simulink model "Integrated_Model"  (R2022a)
settings: Solver=VariableStepAuto  StartTime=0.0  StopTime=10.0  RelTol=1e-3
libraries: simulink x74, simulink_extras x1
settings Model: Creator=user  LastModifiedBy=hp

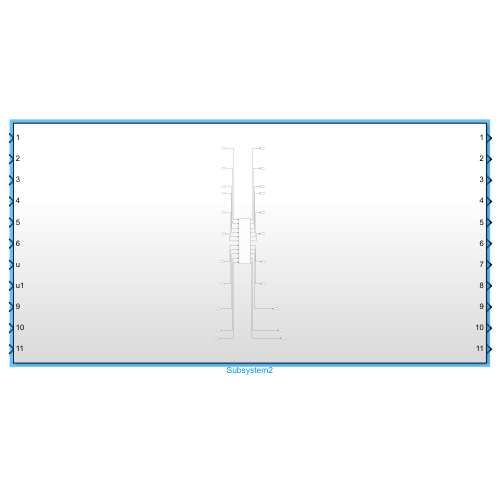
[thumbnail: Simulink's stored preview of the top-level diagram]
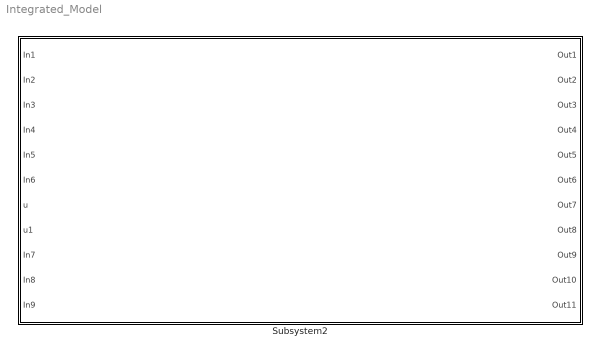
== system Integrated_Model ==
  Subsystem2 : Subsystem

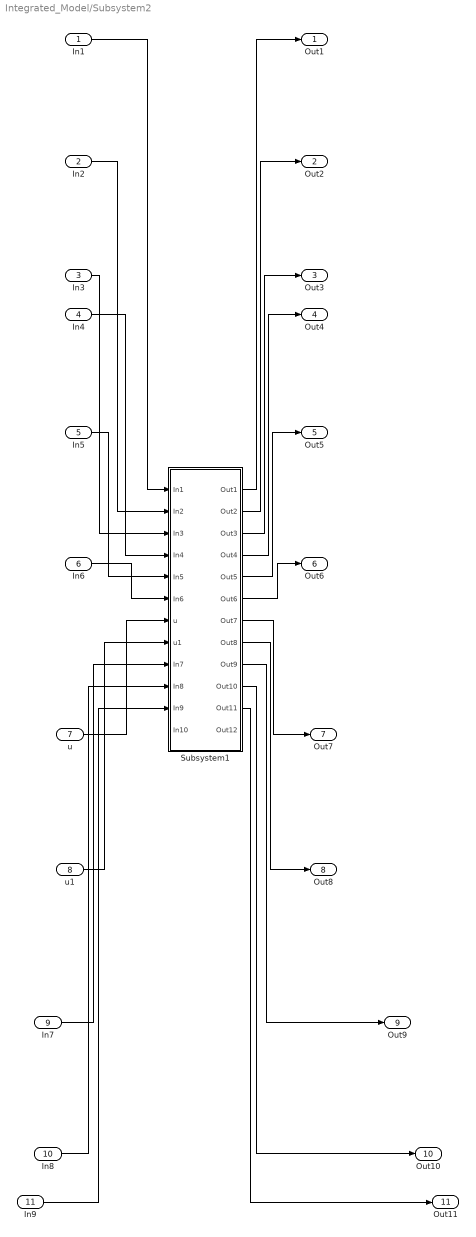
== system Integrated_Model/Subsystem2 ==
  In1 : Inport
  In2 : Inport  Port=2
  In3 : Inport  Port=3
  In4 : Inport  Port=4
  In5 : Inport  Port=5
  In6 : Inport  Port=6
  u : Inport  Port=7
  u1 : Inport  Port=8
  In7 : Inport  Port=9
  In8 : Inport  Port=10
  In9 : Inport  Port=11
  Subsystem1 : Subsystem
  Out1 : Outport
  Out2 : Outport  Port=2
  Out3 : Outport  Port=3
  Out4 : Outport  Port=4
  Out5 : Outport  Port=5
  Out6 : Outport  Port=6
  Out7 : Outport  Port=7
  Out8 : Outport  Port=8
  Out9 : Outport  Port=9
  Out10 : Outport  Port=10
  Out11 : Outport  Port=11
  wires:
  In1/1 -> Subsystem1/1(In1)
  In2/1 -> Subsystem1/2(In2)
  In3/1 -> Subsystem1/3(In3)
  In4/1 -> Subsystem1/4(In4)
  In5/1 -> Subsystem1/5(In5)
  In6/1 -> Subsystem1/6(In6)
  u/1 -> Subsystem1/7(u)
  u1/1 -> Subsystem1/8(u1)
  In7/1 -> Subsystem1/9(In7)
  In8/1 -> Subsystem1/10(In8)
  In9/1 -> Subsystem1/11(In9)
  Subsystem1/1(Out1) -> Out1/1
  Subsystem1/2(Out2) -> Out2/1
  Subsystem1/3(Out3) -> Out3/1
  Subsystem1/4(Out4) -> Out4/1
  Subsystem1/5(Out5) -> Out5/1
  Subsystem1/6(Out6) -> Out6/1
  Subsystem1/7(Out7) -> Out7/1
  Subsystem1/8(Out8) -> Out8/1
  Subsystem1/9(Out9) -> Out9/1
  Subsystem1/10(Out10) -> Out10/1
  Subsystem1/11(Out11) -> Out11/1

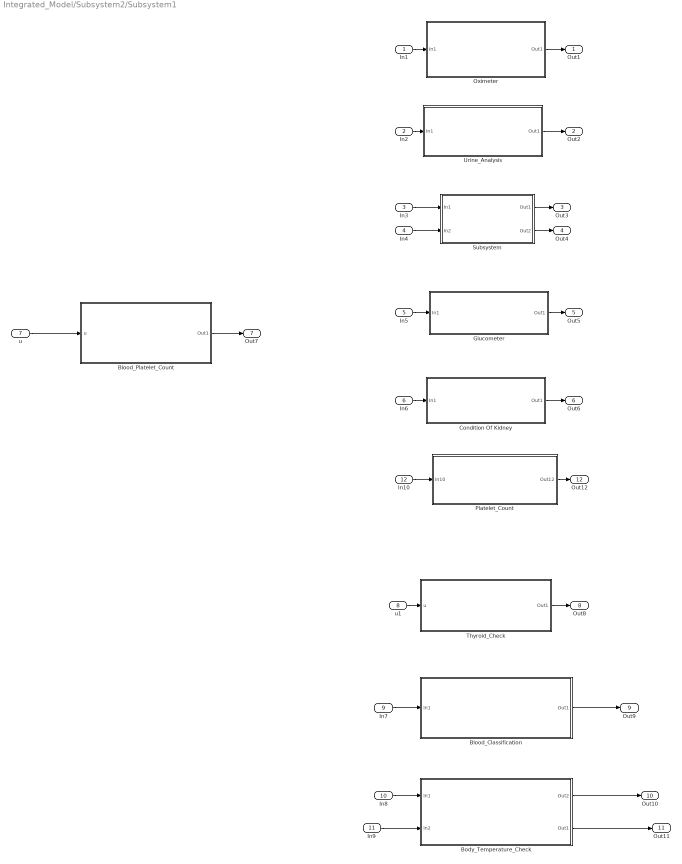
== system Integrated_Model/Subsystem2/Subsystem1 ==
  In1 : Inport
  In2 : Inport  Port=2
  In3 : Inport  Port=3
  In4 : Inport  Port=4
  In5 : Inport  Port=5
  In6 : Inport  Port=6
  u : Inport  Port=7
  u1 : Inport  Port=8
  In7 : Inport  Port=9
  In8 : Inport  Port=10
  In9 : Inport  Port=11
  In10 : Inport  Port=12
  Blood_Classification : Subsystem
  Blood_Platelet_Count : Subsystem
  Body_Temperature_Check : Subsystem
  Condition Of Kidney : Subsystem
  Glucometer : Subsystem
  Oximeter : Subsystem
  Platelet_Count : Subsystem
  Subsystem : Subsystem
  Thyroid_Check : Subsystem
  Urine_Analysis : Subsystem
  Out1 : Outport
  Out2 : Outport  Port=2
  Out3 : Outport  Port=3
  Out4 : Outport  Port=4
  Out5 : Outport  Port=5
  Out6 : Outport  Port=6
  Out7 : Outport  Port=7
  Out8 : Outport  Port=8
  Out9 : Outport  Port=9
  Out10 : Outport  Port=10
  Out11 : Outport  Port=11
  Out12 : Outport  Port=12
  wires:
  In6/1 -> Condition Of Kidney/1(In1)
  Body_Temperature_Check/1(Out2) -> Out10/1
  In8/1 -> Body_Temperature_Check/1(In1)
  In3/1 -> Subsystem/1(In1)
  In4/1 -> Subsystem/2(In2)
  In7/1 -> Blood_Classification/1(In1)
  u1/1 -> Thyroid_Check/1(u)
  In1/1 -> Oximeter/1(In1)
  u/1 -> Blood_Platelet_Count/1(u)
  Urine_Analysis/1(Out1) -> Out2/1
  Subsystem/1(Out1) -> Out3/1
  Subsystem/2(Out2) -> Out4/1
  Oximeter/1(Out1) -> Out1/1
  In2/1 -> Urine_Analysis/1(In1)
  Body_Temperature_Check/2(Out1) -> Out11/1
  Thyroid_Check/1(Out1) -> Out8/1
  Condition Of Kidney/1(Out1) -> Out6/1
  Blood_Classification/1(Out1) -> Out9/1
  Blood_Platelet_Count/1(Out1) -> Out7/1
  In5/1 -> Glucometer/1(In1)
  Glucometer/1(Out1) -> Out5/1
  In9/1 -> Body_Temperature_Check/2(In2)
  In10/1 -> Platelet_Count/1(In10)
  Platelet_Count/1(Out12) -> Out12/1

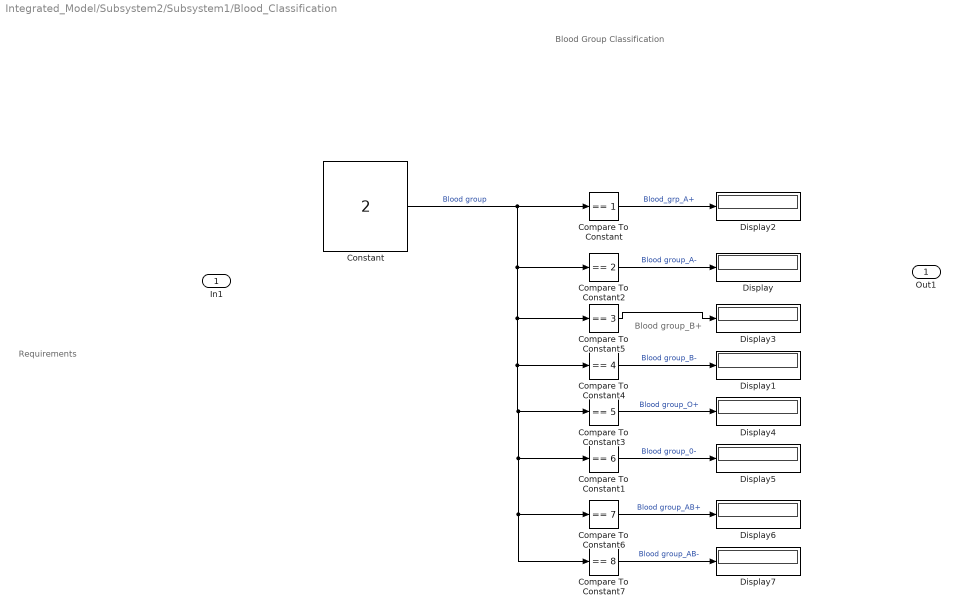
== system Integrated_Model/Subsystem2/Subsystem1/Blood_Classification ==
  note: Requirements
  note: Blood group_B+
  note: Blood Group Classification
  In1 : Inport
  Compare To Constant : simulink/Logic and Bit Operations/Compare To Constant  relop===  const=1  OutDataTypeStr=boolean
  Compare To Constant1 : simulink/Logic and Bit Operations/Compare To Constant  relop===  const=6  OutDataTypeStr=boolean
  Compare To Constant2 : simulink/Logic and Bit Operations/Compare To Constant  relop===  const=2  OutDataTypeStr=boolean
  Compare To Constant3 : simulink/Logic and Bit Operations/Compare To Constant  relop===  const=5  OutDataTypeStr=boolean
  Compare To Constant4 : simulink/Logic and Bit Operations/Compare To Constant  relop===  const=4  OutDataTypeStr=boolean
  Compare To Constant5 : simulink/Logic and Bit Operations/Compare To Constant  relop===  const=3  OutDataTypeStr=boolean
  Compare To Constant6 : simulink/Logic and Bit Operations/Compare To Constant  relop===  const=7  OutDataTypeStr=boolean
  Compare To Constant7 : simulink/Logic and Bit Operations/Compare To Constant  relop===  const=8  OutDataTypeStr=boolean
  Constant : Constant  Value=2
  Display{,1..7} (8 alike) : Display
  Out1 : Outport
  wires:
  Compare To Constant5/1 -> Display3/1
  Compare To Constant4/1 -> Display1/1  "Blood group_B-"
  Constant/1 -> Compare To Constant7/1, Compare To Constant6/1, Compare To Constant1/1, Compare To Constant3/1, Compare To Constant4/1, Compare To Constant5/1, Compare To Constant2/1, Compare To Constant/1  "Blood group"
  Compare To Constant6/1 -> Display6/1  "Blood group_AB+"
  Compare To Constant1/1 -> Display5/1  "Blood group_0-"
  Compare To Constant/1 -> Display2/1  "Blood_grp_A+"
  Compare To Constant2/1 -> Display/1  "Blood group_A-"
  Compare To Constant3/1 -> Display4/1  "Blood group_O+"
  Compare To Constant7/1 -> Display7/1  "Blood group_AB-"

== system Integrated_Model/Subsystem2/Subsystem1/Blood_Platelet_Count ==
  note: BLOOD PLATELET COUNT
  note: INPUTS
      |
      | 0- <150000 Platelets
      | 1- 150000-450000
      | 2- >450000 Platelets
      |
      | OUTPUTS
      | 0 - Thrombocytopenia
      | 1-  Normal
      | 2-  Thrombocytosis
  u : Inport
  Compare To Constant : simulink/Logic and Bit Operations/Compare To Constant  relop===  const=0  OutDataTypeStr=boolean
  Compare To Constant1 : simulink/Logic and Bit Operations/Compare To Constant  relop===  const=1  OutDataTypeStr=boolean
  Compare To Constant2 : simulink/Logic and Bit Operations/Compare To Constant  relop===  const=2  OutDataTypeStr=boolean
  Constant1 : Constant  Value=0
  Constant2 : Constant
  Constant3 : Constant  Value=2
  Constant4 : Constant  Value=2
  Switch : Switch  Criteria=u2 ~= 0  SaturateOnIntegerOverflow=off  InputSameDT=off
  Switch1 : Switch  Criteria=u2 ~= 0  SaturateOnIntegerOverflow=off  InputSameDT=off
  Switch2 : Switch  SaturateOnIntegerOverflow=off  InputSameDT=off
  Out1 : Outport
  wires:
  Switch/1 -> Out1/1
  Constant2/1 -> Switch1/1
  Constant4/1 -> Switch2/3
  Compare To Constant/1 -> Switch/2
  Constant1/1 -> Switch/1
  Compare To Constant2/1 -> Switch2/2
  Compare To Constant1/1 -> Switch1/2
  Switch2/1 -> Switch1/3
  Constant3/1 -> Switch2/1
  Switch1/1 -> Switch/3
  u/1 -> Compare To Constant2/1, Compare To Constant1/1, Compare To Constant/1

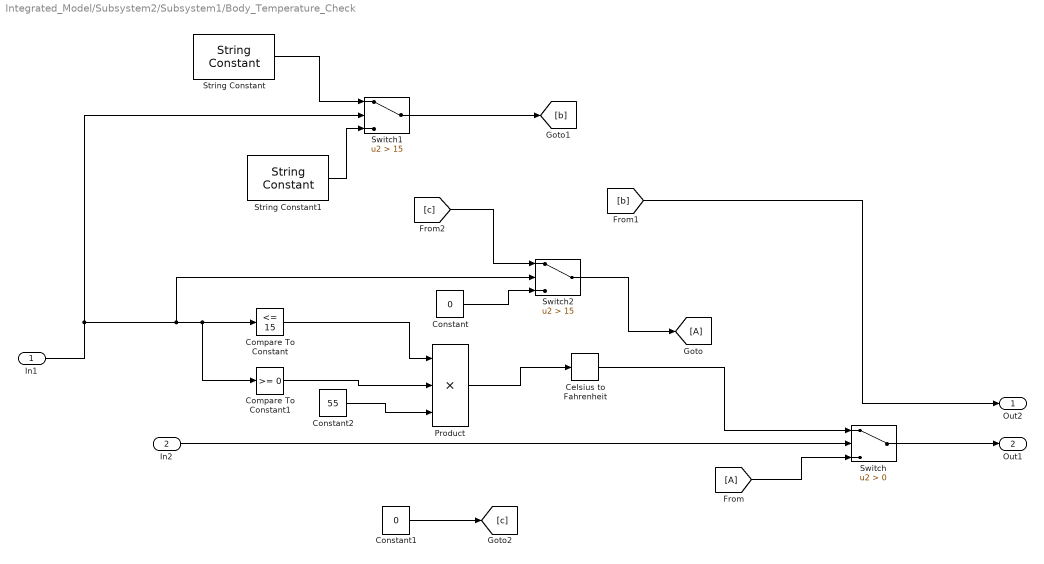
== system Integrated_Model/Subsystem2/Subsystem1/Body_Temperature_Check ==
  In1 : Inport
  In2 : Inport  Port=2
  Celsius to Fahrenheit : simulink_extras/Transformations/Celsius to Fahrenheit
      settings: SourceProductBaseCode=SL
  Compare To Constant : simulink/Logic and Bit Operations/Compare To Constant  relop=<=  const=15  OutDataTypeStr=boolean
  Compare To Constant1 : simulink/Logic and Bit Operations/Compare To Constant  relop=>=  const=0  OutDataTypeStr=boolean
  Constant : Constant  Value=0
  Constant1 : Constant  Value=0
  Constant2 : Constant  Value=55
  From : From
  Goto : Goto
  Product : Product  Inputs=3
  String Constant : StringConstant  String="\"invalid\""
  String Constant1 : StringConstant  String="\"working\""
  Switch : Switch  Criteria=u2 > Threshold  SaturateOnIntegerOverflow=off  InputSameDT=off
  Switch1 : Switch  Criteria=u2 > Threshold  Threshold=15  SaturateOnIntegerOverflow=off  InputSameDT=off
  Switch2 : Switch  Criteria=u2 > Threshold  Threshold=15  SaturateOnIntegerOverflow=off  InputSameDT=off
  Out2 : Outport
  Out1 : Outport  Port=2
  wires:
  Product/1 -> Celsius to Fahrenheit/1
  In2/1 -> Switch/2
  Switch/1 -> Out1/1
  Celsius to Fahrenheit/1 -> Switch/1
  From/1 -> Switch/3
  Constant2/1 -> Product/3
  Compare To Constant/1 -> Product/1
  Compare To Constant1/1 -> Product/2
  String Constant/1 -> Switch1/1
  Switch1/1 -> [b]
  [b] -> Out2/1
  String Constant1/1 -> Switch1/3
  In1/1 -> Switch2/2, Compare To Constant1/1, Compare To Constant/1, Switch1/2
  Switch2/1 -> Goto/1
  Constant/1 -> Switch2/3
  [c] -> Switch2/1
  Constant1/1 -> [c]

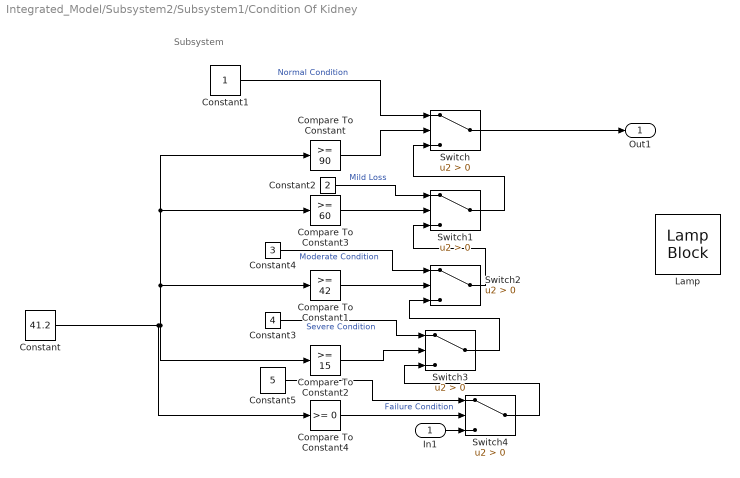
== system Integrated_Model/Subsystem2/Subsystem1/Condition Of Kidney ==
  note: Subsystem
  In1 : Inport
  Compare To Constant : simulink/Logic and Bit Operations/Compare To Constant  relop=>=  const=90  OutDataTypeStr=boolean
  Compare To Constant1 : simulink/Logic and Bit Operations/Compare To Constant  relop=>=  const=42  OutDataTypeStr=boolean
  Compare To Constant2 : simulink/Logic and Bit Operations/Compare To Constant  relop=>=  const=15  OutDataTypeStr=boolean
  Compare To Constant3 : simulink/Logic and Bit Operations/Compare To Constant  relop=>=  const=60  OutDataTypeStr=boolean
  Compare To Constant4 : simulink/Logic and Bit Operations/Compare To Constant  relop=>=  const=0  OutDataTypeStr=boolean
  Constant : Constant  Value=41.2
  Constant1 : Constant
  Constant2 : Constant  Value=2
  Constant3 : Constant  Value=4
  Constant4 : Constant  Value=3
  Constant5 : Constant  Value=5
  Lamp : LampBlock  LabelPosition=Hide
  Switch{,1..4} (5 alike) : Switch  Criteria=u2 > Threshold  SaturateOnIntegerOverflow=off  InputSameDT=off
  Out1 : Outport
  wires:
  Compare To Constant/1 -> Switch/2
  Constant1/1 -> Switch/1  "Normal Condition"
  Compare To Constant4/1 -> Switch4/2
  Switch2/1 -> Switch1/3
  Constant/1 -> Compare To Constant3/1, Compare To Constant/1, Compare To Constant1/1, Compare To Constant2/1, Compare To Constant4/1
  Switch4/1 -> Switch3/3
  Switch1/1 -> Switch/3
  Compare To Constant1/1 -> Switch2/2
  Switch3/1 -> Switch2/3
  Constant3/1 -> Switch3/1  "Severe Condition"
  Constant4/1 -> Switch2/1  "Moderate Condition"
  Compare To Constant2/1 -> Switch3/2
  Compare To Constant3/1 -> Switch1/2
  Constant2/1 -> Switch1/1  "Mild Loss"
  Constant5/1 -> Switch4/1  "Failure Condition"
  In1/1 -> Switch4/3
  Switch/1 -> Out1/1

== system Integrated_Model/Subsystem2/Subsystem1/Glucometer ==
  note: GLUCOMETER
  note: OUTPUTS:
      | 1) Normal
      | 2) Lower PreDiabetes
      | 3) Higher PreDiabetes
      | 4) Light Dehydrated
      | 5) Symptomatic Diabetes
      | 6) High Risk
  note: REQUIREMENT INPUT:
      |
      | Below 5.7% is normal.
      | 5.7% to 6.4% is diagnosed as prediabetes.
      | 6.5% or higher on two separate tests indicates diabetes.
      | Name - Yash Rastogi
      | PS.NO. - 99007892
      | Team J
  In1 : Inport
  Constant : Constant  Value=5.8
  Display : Display
  Subsystem : Subsystem
  Out1 : Outport
  wires:
  Constant/1 -> Subsystem/1(In1)
  Subsystem/1(Out1) -> Display/1

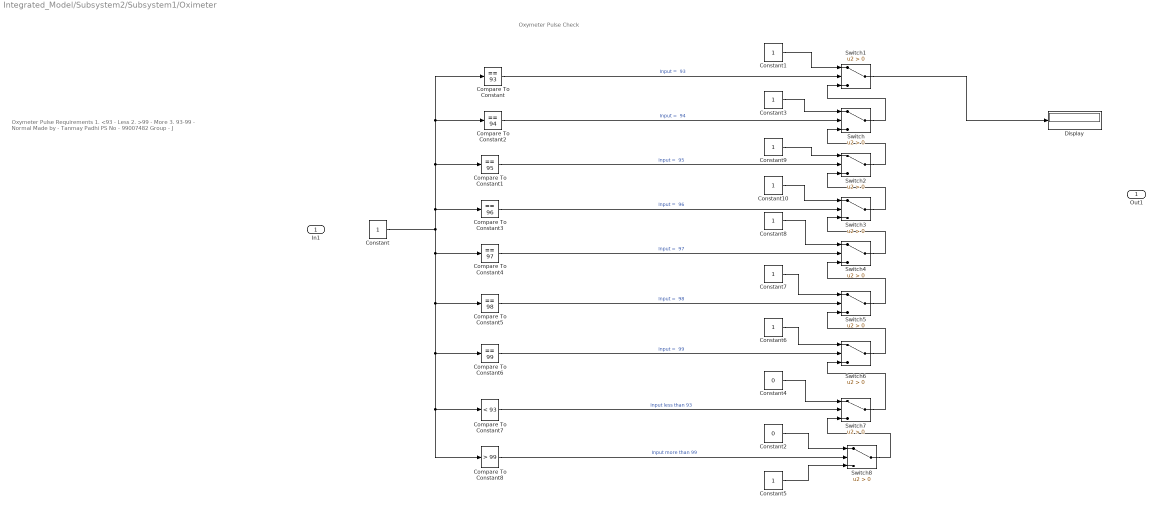
== system Integrated_Model/Subsystem2/Subsystem1/Oximeter ==
  note: Oxymeter Pulse
      |
      | Requirements
      | 1. <93 - Less
      | 2. >99 - More
      | 3. 93-99 - Normal
      |
      | Made by - Tanmay Padhi
      | PS No - 99007482
      | Group - J
  note: Oxymeter Pulse Check
  In1 : Inport
  Compare To Constant : simulink/Logic and Bit Operations/Compare To Constant  relop===  const=93  OutDataTypeStr=boolean
  Compare To Constant1 : simulink/Logic and Bit Operations/Compare To Constant  relop===  const=95  OutDataTypeStr=boolean
  Compare To Constant2 : simulink/Logic and Bit Operations/Compare To Constant  relop===  const=94  OutDataTypeStr=boolean
  Compare To Constant3 : simulink/Logic and Bit Operations/Compare To Constant  relop===  const=96  OutDataTypeStr=boolean
  Compare To Constant4 : simulink/Logic and Bit Operations/Compare To Constant  relop===  const=97  OutDataTypeStr=boolean
  Compare To Constant5 : simulink/Logic and Bit Operations/Compare To Constant  relop===  const=98  OutDataTypeStr=boolean
  Compare To Constant6 : simulink/Logic and Bit Operations/Compare To Constant  relop===  const=99  OutDataTypeStr=boolean
  Compare To Constant7 : simulink/Logic and Bit Operations/Compare To Constant  relop=<  const=93  OutDataTypeStr=boolean
  Compare To Constant8 : simulink/Logic and Bit Operations/Compare To Constant  relop=>  const=99  OutDataTypeStr=boolean
  Constant{,1,3,5..10} (9 alike) : Constant
  Constant2 : Constant  Value=0
  Constant4 : Constant  Value=0
  Display : Display
  Switch{,1..8} (9 alike) : Switch  Criteria=u2 > Threshold  SaturateOnIntegerOverflow=off  InputSameDT=off
  Out1 : Outport
  wires:
  Switch7/1 -> Switch6/3
  Compare To Constant4/1 -> Switch4/2  "Input =  97"
  Constant1/1 -> Switch1/1
  Compare To Constant7/1 -> Switch7/2  "Input less than 93"
  Switch6/1 -> Switch5/3
  Constant/1 -> Compare To Constant4/1, Compare To Constant5/1, Compare To Constant8/1, Compare To Constant7/1, Compare To Constant6/1, Compare To Constant2/1, Compare To Constant/1, Compare To Constant1/1, Compare To Constant3/1
  Compare To Constant5/1 -> Switch5/2  "Input =  98"
  Switch4/1 -> Switch3/3
  Constant9/1 -> Switch2/1
  Compare To Constant/1 -> Switch1/2  "Input =  93"
  Compare To Constant1/1 -> Switch2/2  "Input =  95"
  Constant5/1 -> Switch8/3
  Constant3/1 -> Switch/1
  Switch3/1 -> Switch2/3
  Switch2/1 -> Switch/3
  Constant8/1 -> Switch4/1
  Compare To Constant3/1 -> Switch3/2  "Input =  96"
  Switch/1 -> Switch1/3
  Compare To Constant8/1 -> Switch8/2  "Input more than 99"
  Constant6/1 -> Switch6/1
  Constant4/1 -> Switch7/1
  Switch8/1 -> Switch7/3
  Constant7/1 -> Switch5/1
  Compare To Constant6/1 -> Switch6/2  "Input =  99"
  Switch5/1 -> Switch4/3
  Compare To Constant2/1 -> Switch/2  "Input =  94"
  Constant2/1 -> Switch8/1
  Constant10/1 -> Switch3/1
  Switch1/1 -> Display/1

== system Integrated_Model/Subsystem2/Subsystem1/Platelet_Count ==
  note: INPUTS
      |
      | 0- <150000 Platelets
      | 1- 150000-450000
      | 2- >450000 Platelets
      |
      | OUTPUTS
      | 0 - Thrombocytopenia
      | 1-  Normal
      | 2-  Thrombocytosis
  note: BLOOD PLATELET COUNT
  In10 : Inport
  AND : Logic  Inputs=3  IconShape=distinctive  AllPortsSameDT=off  OutDataTypeStr=boolean
  Display : Display
  Subsystem1 : Subsystem
  Subsystem2 : Subsystem
  Subsystem3 : Subsystem
  Out12 : Outport
  wires:
  Subsystem1/1(Out2) -> Out12/1
  AND/1 -> Display/1
  Subsystem3/1(Out1) -> AND/3
  Subsystem2/1(Out1) -> AND/2
  In10/1 -> Subsystem1/1(In1)
  Subsystem1/2(Out1) -> AND/1

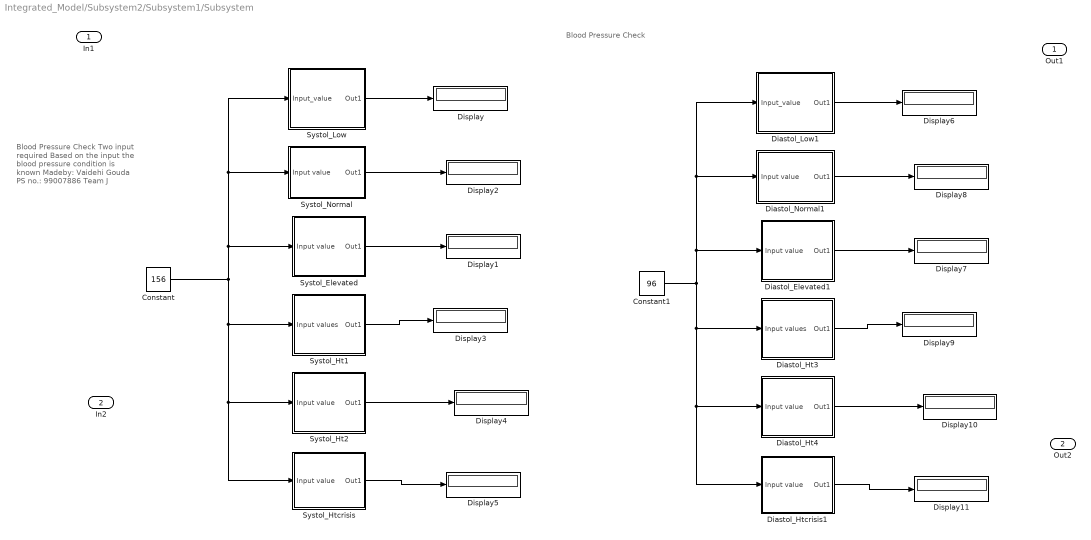
== system Integrated_Model/Subsystem2/Subsystem1/Subsystem ==
  note: Blood Pressure Check
      |
      | Two input required
      | Based on the input the blood pressure condition is known
      |
      | Madeby: Vaidehi Gouda
      | PS no.: 99007886
      | Team J
  note: Blood Pressure Check
  In1 : Inport
  In2 : Inport  Port=2
  Constant : Constant  Value=156
  Constant1 : Constant  Value=96
  Diastol_Elevated1 : Subsystem
  Diastol_Ht3 : Subsystem
  Diastol_Ht4 : Subsystem
  Diastol_Htcrisis1 : Subsystem
  Diastol_Low1 : Subsystem
  Diastol_Normal1 : Subsystem
  Display{,1..11} (12 alike) : Display
  Systol_Elevated : Subsystem
  Systol_Ht1 : Subsystem
  Systol_Ht2 : Subsystem
  Systol_Htcrisis : Subsystem
  Systol_Low : Subsystem
  Systol_Normal : Subsystem
  Out1 : Outport
  Out2 : Outport  Port=2
  wires:
  Constant1/1 -> Diastol_Elevated1/1(Input value), Diastol_Normal1/1(Input value), Diastol_Low1/1(Input_value), Diastol_Ht3/1(Input values), Diastol_Ht4/1(Input value), Diastol_Htcrisis1/1(Input value)
  Diastol_Htcrisis1/1(Out1) -> Display11/1
  Systol_Ht1/1(Out1) -> Display3/1
  Systol_Normal/1(Out1) -> Display2/1
  Systol_Elevated/1(Out1) -> Display1/1
  Constant/1 -> Systol_Htcrisis/1(Input value), Systol_Ht2/1(Input value), Systol_Ht1/1(Input values), Systol_Low/1(Input_value), Systol_Normal/1(Input value), Systol_Elevated/1(Input value)
  Systol_Ht2/1(Out1) -> Display4/1
  Diastol_Ht3/1(Out1) -> Display9/1
  Diastol_Elevated1/1(Out1) -> Display7/1
  Systol_Htcrisis/1(Out1) -> Display5/1
  Diastol_Normal1/1(Out1) -> Display8/1
  Diastol_Low1/1(Out1) -> Display6/1
  Diastol_Ht4/1(Out1) -> Display10/1
  Systol_Low/1(Out1) -> Display/1

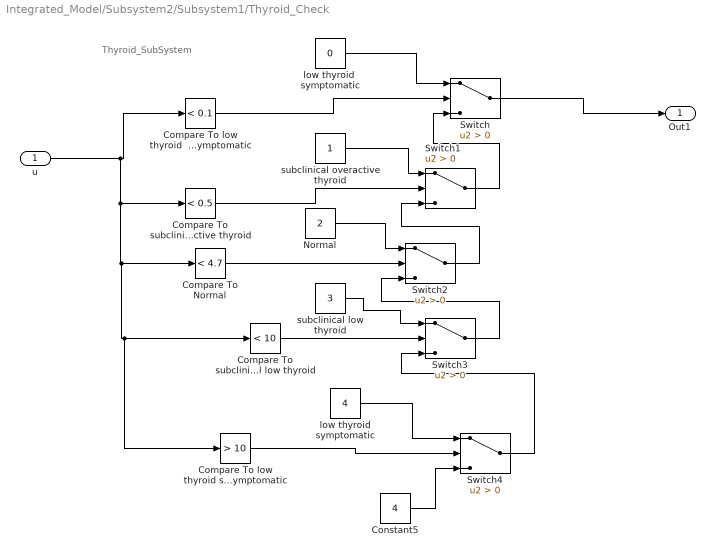
== system Integrated_Model/Subsystem2/Subsystem1/Thyroid_Check ==
  note: Thyroid_SubSystem
  u : Inport
  Compare To Normal : simulink/Logic and Bit Operations/Compare To Constant  relop=<  const=4.7  OutDataTypeStr=boolean
  Compare To low thyroid  symptomatic : simulink/Logic and Bit Operations/Compare To Constant  relop=<  const=0.1  OutDataTypeStr=boolean
  Compare To low thyroid symptomatic : simulink/Logic and Bit Operations/Compare To Constant  relop=>  const=10  OutDataTypeStr=boolean
  "Compare To subclinical low thyroid " : simulink/Logic and Bit Operations/Compare To Constant  relop=<  const=10  OutDataTypeStr=boolean
  Compare To subclinical overactive thyroid : simulink/Logic and Bit Operations/Compare To Constant  relop=<  const=0.5  OutDataTypeStr=boolean
  Constant5 : Constant  Value=4
  Normal : Constant  Value=2
  Switch{,1..4} (5 alike) : Switch  Criteria=u2 > Threshold  SaturateOnIntegerOverflow=off  InputSameDT=off
  low thyroid  symptomatic : Constant  Value=0
  low thyroid symptomatic : Constant  Value=4
  subclinical low thyroid : Constant  Value=3
  subclinical overactive thyroid : Constant
  Out1 : Outport
  wires:
  Compare To low thyroid  symptomatic/1 -> Switch/2
  Switch/1 -> Out1/1
  low thyroid  symptomatic/1 -> Switch/1
  Constant5/1 -> Switch4/3
  Switch3/1 -> Switch2/3
  u/1 -> Compare To low thyroid symptomatic/1, "Compare To subclinical low thyroid "/1, Compare To Normal/1, Compare To subclinical overactive thyroid/1, Compare To low thyroid  symptomatic/1
  "Compare To subclinical low thyroid "/1 -> Switch3/2
  Switch1/1 -> Switch/3
  Compare To low thyroid symptomatic/1 -> Switch4/2
  Switch4/1 -> Switch3/3
  Normal/1 -> Switch2/1
  Switch2/1 -> Switch1/3
  Compare To subclinical overactive thyroid/1 -> Switch1/2
  low thyroid symptomatic/1 -> Switch4/1
  subclinical low thyroid/1 -> Switch3/1
  Compare To Normal/1 -> Switch2/2
  subclinical overactive thyroid/1 -> Switch1/1

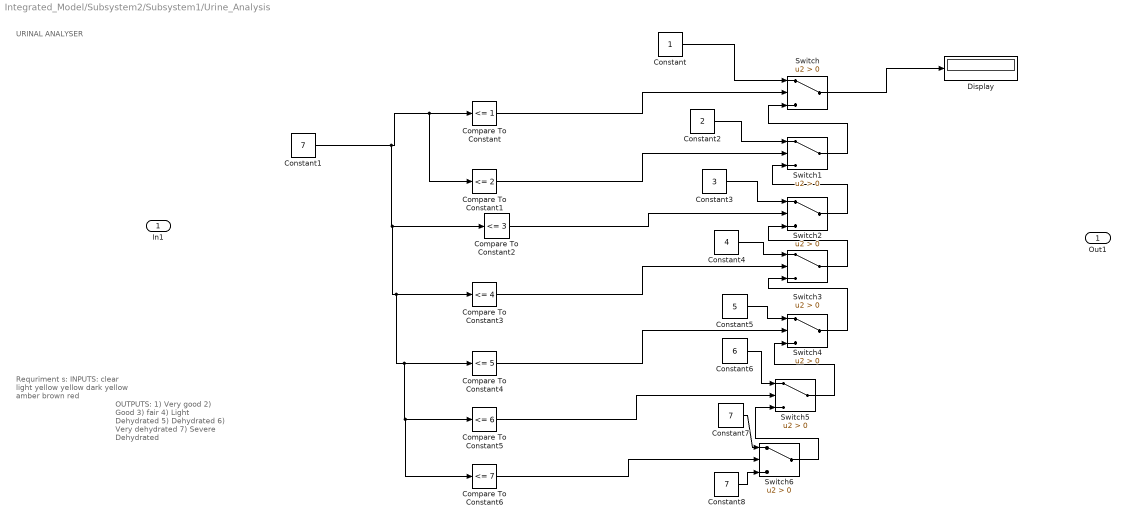
== system Integrated_Model/Subsystem2/Subsystem1/Urine_Analysis ==
  note: OUTPUTS:
      |  1) Very good
      | 2) Good
      | 3) fair
      | 4) Light Dehydrated
      | 5) Dehydrated
      | 6) Very dehydrated
      | 7) Severe Dehydrated
  note: Requriment s:
      | INPUTS:
      | clear
      | light yellow
      | yellow
      | dark yellow
      | amber
      | brown
      | red
  note: URINAL ANALYSER
  In1 : Inport
  Compare To Constant : simulink/Logic and Bit Operations/Compare To Constant  relop=<=  const=1  OutDataTypeStr=boolean
  Compare To Constant1 : simulink/Logic and Bit Operations/Compare To Constant  relop=<=  const=2  OutDataTypeStr=boolean
  Compare To Constant2 : simulink/Logic and Bit Operations/Compare To Constant  relop=<=  const=3  OutDataTypeStr=boolean
  Compare To Constant3 : simulink/Logic and Bit Operations/Compare To Constant  relop=<=  const=4  OutDataTypeStr=boolean
  Compare To Constant4 : simulink/Logic and Bit Operations/Compare To Constant  relop=<=  const=5  OutDataTypeStr=boolean
  Compare To Constant5 : simulink/Logic and Bit Operations/Compare To Constant  relop=<=  const=6  OutDataTypeStr=boolean
  Compare To Constant6 : simulink/Logic and Bit Operations/Compare To Constant  relop=<=  const=7  OutDataTypeStr=boolean
  Constant : Constant
  Constant1 : Constant  Value=7
  Constant2 : Constant  Value=2
  Constant3 : Constant  Value=3
  Constant4 : Constant  Value=4
  Constant5 : Constant  Value=5
  Constant6 : Constant  Value=6
  Constant7 : Constant  Value=7
  Constant8 : Constant  Value=7
  Display : Display
  Switch{,1..6} (7 alike) : Switch  Criteria=u2 > Threshold  SaturateOnIntegerOverflow=off  InputSameDT=off
  Out1 : Outport
  wires:
  Constant/1 -> Switch/1
  Constant1/1 -> Compare To Constant6/1, Compare To Constant5/1, Compare To Constant4/1, Compare To Constant3/1, Compare To Constant2/1, Compare To Constant1/1, Compare To Constant/1
  Constant2/1 -> Switch1/1
  Compare To Constant5/1 -> Switch5/2
  Compare To Constant2/1 -> Switch2/2
  Compare To Constant/1 -> Switch/2
  Compare To Constant1/1 -> Switch1/2
  Constant5/1 -> Switch4/1
  Constant6/1 -> Switch5/1
  Switch6/1 -> Switch5/3
  Switch2/1 -> Switch1/3
  Switch4/1 -> Switch3/3
  Compare To Constant4/1 -> Switch4/2
  Switch1/1 -> Switch/3
  Constant4/1 -> Switch3/1
  Switch3/1 -> Switch2/3
  Compare To Constant3/1 -> Switch3/2
  Switch/1 -> Display/1
  Compare To Constant6/1 -> Switch6/2
  Constant3/1 -> Switch2/1
  Switch5/1 -> Switch4/3
  Constant8/1 -> Switch6/3
  Constant7/1 -> Switch6/1

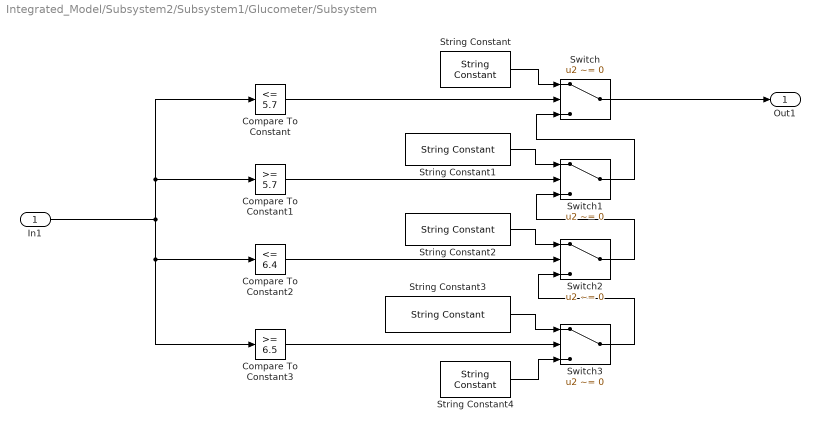
== system Integrated_Model/Subsystem2/Subsystem1/Glucometer/Subsystem ==
  In1 : Inport
  Compare To Constant : simulink/Logic and Bit Operations/Compare To Constant  relop=<=  const=5.7  OutDataTypeStr=boolean
  Compare To Constant1 : simulink/Logic and Bit Operations/Compare To Constant  relop=>=  const=5.7  OutDataTypeStr=boolean
  Compare To Constant2 : simulink/Logic and Bit Operations/Compare To Constant  relop=<=  const=6.4  OutDataTypeStr=boolean
  Compare To Constant3 : simulink/Logic and Bit Operations/Compare To Constant  relop=>=  const=6.5  OutDataTypeStr=boolean
  String Constant : StringConstant  String="\"Normal\""
  String Constant1 : StringConstant  String="\"Lower PreDiabetes\""
  String Constant2 : StringConstant  String="\"Higher PreDiabetes\""
  String Constant3 : StringConstant  String="\"Symptomatic Diabetes\""
  String Constant4 : StringConstant  String="\"High Risk\""
  Switch{,1..3} (4 alike) : Switch  Criteria=u2 ~= 0  SaturateOnIntegerOverflow=off  InputSameDT=off
  Out1 : Outport
  wires:
  In1/1 -> Compare To Constant3/1, Compare To Constant2/1, Compare To Constant1/1, Compare To Constant/1
  Switch2/1 -> Switch1/3
  String Constant4/1 -> Switch3/3
  Compare To Constant3/1 -> Switch3/2
  Switch3/1 -> Switch2/3
  Compare To Constant2/1 -> Switch2/2
  Switch1/1 -> Switch/3
  Compare To Constant/1 -> Switch/2
  Compare To Constant1/1 -> Switch1/2
  String Constant2/1 -> Switch2/1
  Switch/1 -> Out1/1
  String Constant1/1 -> Switch1/1
  String Constant/1 -> Switch/1
  String Constant3/1 -> Switch3/1

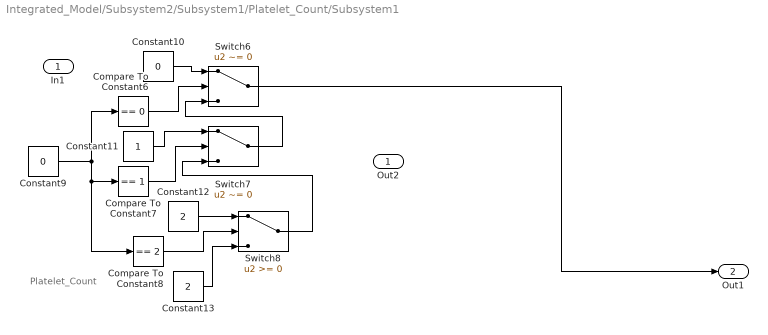
== system Integrated_Model/Subsystem2/Subsystem1/Platelet_Count/Subsystem1 ==
  note: Platelet_Count
  In1 : Inport
  Compare To Constant6 : simulink/Logic and Bit Operations/Compare To Constant  relop===  const=0  OutDataTypeStr=boolean
  Compare To Constant7 : simulink/Logic and Bit Operations/Compare To Constant  relop===  const=1  OutDataTypeStr=boolean
  Compare To Constant8 : simulink/Logic and Bit Operations/Compare To Constant  relop===  const=2  OutDataTypeStr=boolean
  Constant10 : Constant  Value=0
  Constant11 : Constant
  Constant12 : Constant  Value=2
  Constant13 : Constant  Value=2
  Constant9 : Constant  Value=0
  Switch6 : Switch  Criteria=u2 ~= 0  SaturateOnIntegerOverflow=off  InputSameDT=off
  Switch7 : Switch  Criteria=u2 ~= 0  SaturateOnIntegerOverflow=off  InputSameDT=off
  Switch8 : Switch  SaturateOnIntegerOverflow=off  InputSameDT=off
  Out2 : Outport
  Out1 : Outport  Port=2
  wires:
  Constant11/1 -> Switch7/1
  Compare To Constant6/1 -> Switch6/2
  Switch6/1 -> Out1/1
  Constant9/1 -> Compare To Constant6/1, Compare To Constant8/1, Compare To Constant7/1
  Switch8/1 -> Switch7/3
  Constant10/1 -> Switch6/1
  Compare To Constant7/1 -> Switch7/2
  Switch7/1 -> Switch6/3
  Constant13/1 -> Switch8/3
  Constant12/1 -> Switch8/1
  Compare To Constant8/1 -> Switch8/2

== system Integrated_Model/Subsystem2/Subsystem1/Platelet_Count/Subsystem2 ==
  note: Red_Blood_cell
  Compare To Constant3 : simulink/Logic and Bit Operations/Compare To Constant  relop===  const=0  OutDataTypeStr=boolean
  Compare To Constant4 : simulink/Logic and Bit Operations/Compare To Constant  relop===  const=1  OutDataTypeStr=boolean
  Compare To Constant5 : simulink/Logic and Bit Operations/Compare To Constant  relop===  const=2  OutDataTypeStr=boolean
  Constant : Constant
  Constant5 : Constant  Value=0
  Constant6 : Constant
  Constant7 : Constant  Value=2
  Constant8 : Constant  Value=2
  Switch3 : Switch  Criteria=u2 ~= 0  SaturateOnIntegerOverflow=off  InputSameDT=off
  Switch4 : Switch  Criteria=u2 ~= 0  SaturateOnIntegerOverflow=off  InputSameDT=off
  Switch5 : Switch  SaturateOnIntegerOverflow=off  InputSameDT=off
  Out1 : Outport
  wires:
  Switch4/1 -> Switch3/3
  Compare To Constant4/1 -> Switch4/2
  Constant6/1 -> Switch4/1
  Switch5/1 -> Switch4/3
  Constant5/1 -> Switch3/1
  Constant8/1 -> Switch5/3
  Compare To Constant5/1 -> Switch5/2
  Constant7/1 -> Switch5/1
  Compare To Constant3/1 -> Switch3/2
  Constant/1 -> Compare To Constant3/1, Compare To Constant5/1, Compare To Constant4/1
  Switch3/1 -> Out1/1

== system Integrated_Model/Subsystem2/Subsystem1/Platelet_Count/Subsystem3 ==
  note: White_Blood_cell
  Compare To Constant1 : simulink/Logic and Bit Operations/Compare To Constant  relop===  const=0  OutDataTypeStr=boolean
  Compare To Constant2 : simulink/Logic and Bit Operations/Compare To Constant  relop===  const=1  OutDataTypeStr=boolean
  Compare To Constant9 : simulink/Logic and Bit Operations/Compare To Constant  relop===  const=2  OutDataTypeStr=boolean
  Constant1 : Constant
  Constant14 : Constant  Value=2
  Constant2 : Constant  Value=0
  Constant3 : Constant
  Constant4 : Constant  Value=2
  Switch1 : Switch  Criteria=u2 ~= 0  SaturateOnIntegerOverflow=off  InputSameDT=off
  Switch2 : Switch  Criteria=u2 ~= 0  SaturateOnIntegerOverflow=off  InputSameDT=off
  Switch9 : Switch  SaturateOnIntegerOverflow=off  InputSameDT=off
  Out1 : Outport
  wires:
  Constant1/1 -> Compare To Constant1/1, Compare To Constant9/1, Compare To Constant2/1
  Compare To Constant9/1 -> Switch9/2
  Switch9/1 -> Switch2/3
  Constant14/1 -> Switch9/3
  Constant2/1 -> Switch1/1
  Constant4/1 -> Switch9/1
  Compare To Constant1/1 -> Switch1/2
  Constant3/1 -> Switch2/1
  Switch2/1 -> Switch1/3
  Compare To Constant2/1 -> Switch2/2
  Switch1/1 -> Out1/1

== system Integrated_Model/Subsystem2/Subsystem1/Subsystem/Diastol_Elevated1 ==
  Input value : Inport
  121+Compare : simulink/Logic and Bit Operations/Compare To Constant  relop=>  const=75  OutDataTypeStr=boolean
  129-Compare : simulink/Logic and Bit Operations/Compare To Constant  relop=<=  const=80  OutDataTypeStr=boolean
  Constant25 : Constant  Value=3
  Constant5 : Constant
  Constant6 : Constant
  Constant7 : Constant  Value=0
  Constant8 : Constant  Value=0
  Logical Operator1 : Logic  AllPortsSameDT=off  OutDataTypeStr=boolean
  Product2 : Product
  Range_Lower : Switch  Criteria=u2 > Threshold  SaturateOnIntegerOverflow=off  InputSameDT=off
  Range_Upper : Switch  Criteria=u2 > Threshold  SaturateOnIntegerOverflow=off  InputSameDT=off
  Out1 : Outport
  wires:
  Logical Operator1/1 -> Product2/1
  Constant7/1 -> Range_Upper/3
  Input value/1 -> 129-Compare/1, 121+Compare/1
  Product2/1 -> Out1/1
  Constant6/1 -> Range_Lower/1
  Constant8/1 -> Range_Lower/3
  Constant25/1 -> Product2/2
  Constant5/1 -> Range_Upper/1
  121+Compare/1 -> Range_Upper/2
  Range_Upper/1 -> Logical Operator1/1
  129-Compare/1 -> Range_Lower/2
  Range_Lower/1 -> Logical Operator1/2

== system Integrated_Model/Subsystem2/Subsystem1/Subsystem/Diastol_Ht3 ==
  Input values : Inport
  130+Compare : simulink/Logic and Bit Operations/Compare To Constant  relop=>  const=80  OutDataTypeStr=boolean
  139-Compare : simulink/Logic and Bit Operations/Compare To Constant  relop=<=  const=89  OutDataTypeStr=boolean
  Constant11 : Constant
  Constant12 : Constant
  Constant13 : Constant  Value=0
  Constant14 : Constant  Value=0
  Constant26 : Constant  Value=4
  Logical Operator2 : Logic  AllPortsSameDT=off  OutDataTypeStr=boolean
  Product3 : Product
  Range_Lower : Switch  Criteria=u2 > Threshold  SaturateOnIntegerOverflow=off  InputSameDT=off
  Range_Upper : Switch  Criteria=u2 > Threshold  SaturateOnIntegerOverflow=off  InputSameDT=off
  Out1 : Outport
  wires:
  Constant13/1 -> Range_Upper/3
  Range_Upper/1 -> Logical Operator2/1
  Product3/1 -> Out1/1
  Range_Lower/1 -> Logical Operator2/2
  139-Compare/1 -> Range_Lower/2
  130+Compare/1 -> Range_Upper/2
  Logical Operator2/1 -> Product3/1
  Constant12/1 -> Range_Lower/1
  Constant14/1 -> Range_Lower/3
  Constant11/1 -> Range_Upper/1
  Constant26/1 -> Product3/2
  Input values/1 -> 130+Compare/1, 139-Compare/1

== system Integrated_Model/Subsystem2/Subsystem1/Subsystem/Diastol_Ht4 ==
  Input value : Inport
  140+Compare : simulink/Logic and Bit Operations/Compare To Constant  relop=>=  const=90  OutDataTypeStr=boolean
  159-Compare : simulink/Logic and Bit Operations/Compare To Constant  relop=<=  const=99  OutDataTypeStr=boolean
  Constant15 : Constant
  Constant16 : Constant
  Constant17 : Constant  Value=0
  Constant18 : Constant  Value=0
  Constant27 : Constant  Value=5
  Logical Operator3 : Logic  AllPortsSameDT=off  OutDataTypeStr=boolean
  Product4 : Product
  Range_Lower : Switch  Criteria=u2 > Threshold  SaturateOnIntegerOverflow=off  InputSameDT=off
  Range_Upper : Switch  Criteria=u2 > Threshold  SaturateOnIntegerOverflow=off  InputSameDT=off
  Out1 : Outport
  wires:
  Product4/1 -> Out1/1
  Constant15/1 -> Range_Upper/1
  140+Compare/1 -> Range_Upper/2
  Logical Operator3/1 -> Product4/1
  Constant18/1 -> Range_Lower/3
  Range_Lower/1 -> Logical Operator3/2
  Range_Upper/1 -> Logical Operator3/1
  Input value/1 -> 159-Compare/1, 140+Compare/1
  Constant17/1 -> Range_Upper/3
  Constant27/1 -> Product4/2
  159-Compare/1 -> Range_Lower/2
  Constant16/1 -> Range_Lower/1

== system Integrated_Model/Subsystem2/Subsystem1/Subsystem/Diastol_Htcrisis1 ==
  Input value : Inport
  180+Compare : simulink/Logic and Bit Operations/Compare To Constant  relop=>=  const=120  OutDataTypeStr=boolean
  260-Compare : simulink/Logic and Bit Operations/Compare To Constant  relop=<=  const=170  OutDataTypeStr=boolean
  Constant19 : Constant
  Constant20 : Constant
  Constant21 : Constant  Value=0
  Constant22 : Constant  Value=0
  Constant28 : Constant  Value=6
  Logical Operator4 : Logic  AllPortsSameDT=off  OutDataTypeStr=boolean
  Product5 : Product
  Range_Lower : Switch  Criteria=u2 > Threshold  SaturateOnIntegerOverflow=off  InputSameDT=off
  Range_Upper : Switch  Criteria=u2 > Threshold  SaturateOnIntegerOverflow=off  InputSameDT=off
  Out1 : Outport
  wires:
  Product5/1 -> Out1/1
  Input value/1 -> 260-Compare/1, 180+Compare/1
  Constant19/1 -> Range_Upper/1
  Constant28/1 -> Product5/2
  Logical Operator4/1 -> Product5/1
  Range_Upper/1 -> Logical Operator4/1
  Constant20/1 -> Range_Lower/1
  180+Compare/1 -> Range_Upper/2
  260-Compare/1 -> Range_Lower/2
  Constant22/1 -> Range_Lower/3
  Constant21/1 -> Range_Upper/3
  Range_Lower/1 -> Logical Operator4/2

== system Integrated_Model/Subsystem2/Subsystem1/Subsystem/Diastol_Low1 ==
  Input_value : Inport
  100-Compare : simulink/Logic and Bit Operations/Compare To Constant  relop=<=  const=74  OutDataTypeStr=boolean
  90+compare : simulink/Logic and Bit Operations/Compare To Constant  relop=>=  const=60  OutDataTypeStr=boolean
  Constant1 : Constant
  Constant2 : Constant
  Constant23 : Constant
  Constant3 : Constant  Value=0
  Constant4 : Constant  Value=0
  Logical Operator : Logic  AllPortsSameDT=off  OutDataTypeStr=boolean
  Product : Product
  Range_Lower : Switch  Criteria=u2 > Threshold  SaturateOnIntegerOverflow=off  InputSameDT=off
  Range_Upper : Switch  Criteria=u2 > Threshold  SaturateOnIntegerOverflow=off  InputSameDT=off
  Out1 : Outport
  wires:
  Product/1 -> Out1/1
  Constant2/1 -> Range_Lower/1
  Constant4/1 -> Range_Lower/3
  90+compare/1 -> Range_Upper/2
  100-Compare/1 -> Range_Lower/2
  Range_Upper/1 -> Logical Operator/1
  Constant23/1 -> Product/2
  Constant1/1 -> Range_Upper/1
  Range_Lower/1 -> Logical Operator/2
  Input_value/1 -> 90+compare/1, 100-Compare/1
  Constant3/1 -> Range_Upper/3
  Logical Operator/1 -> Product/1

== system Integrated_Model/Subsystem2/Subsystem1/Subsystem/Diastol_Normal1 ==
  Input value : Inport
  120Compare : simulink/Logic and Bit Operations/Compare To Constant  relop===  const=80  OutDataTypeStr=boolean
  Constant10 : Constant  Value=0
  Constant24 : Constant  Value=2
  Constant9 : Constant
  Product1 : Product
  Range_compare : Switch  Criteria=u2 > Threshold  SaturateOnIntegerOverflow=off  InputSameDT=off
  Out1 : Outport
  wires:
  Constant10/1 -> Range_compare/3
  Input value/1 -> 120Compare/1
  Product1/1 -> Out1/1
  Constant24/1 -> Product1/2
  Range_compare/1 -> Product1/1
  120Compare/1 -> Range_compare/2
  Constant9/1 -> Range_compare/1

== system Integrated_Model/Subsystem2/Subsystem1/Subsystem/Systol_Elevated ==
  Input value : Inport
  121+Compare : simulink/Logic and Bit Operations/Compare To Constant  relop=>=  const=121  OutDataTypeStr=boolean
  129-Compare : simulink/Logic and Bit Operations/Compare To Constant  relop=<=  const=129  OutDataTypeStr=boolean
  Constant25 : Constant  Value=3
  Constant5 : Constant
  Constant6 : Constant
  Constant7 : Constant  Value=0
  Constant8 : Constant  Value=0
  Logical Operator1 : Logic  AllPortsSameDT=off  OutDataTypeStr=boolean
  Product2 : Product
  Range_Lower : Switch  Criteria=u2 > Threshold  SaturateOnIntegerOverflow=off  InputSameDT=off
  Range_Upper : Switch  Criteria=u2 > Threshold  SaturateOnIntegerOverflow=off  InputSameDT=off
  Out1 : Outport
  wires:
  Range_Lower/1 -> Logical Operator1/2
  129-Compare/1 -> Range_Lower/2
  Range_Upper/1 -> Logical Operator1/1
  121+Compare/1 -> Range_Upper/2
  Constant5/1 -> Range_Upper/1
  Constant25/1 -> Product2/2
  Constant8/1 -> Range_Lower/3
  Constant6/1 -> Range_Lower/1
  Product2/1 -> Out1/1
  Input value/1 -> 121+Compare/1, 129-Compare/1
  Constant7/1 -> Range_Upper/3
  Logical Operator1/1 -> Product2/1

== system Integrated_Model/Subsystem2/Subsystem1/Subsystem/Systol_Ht1 ==
  Input values : Inport
  130+Compare : simulink/Logic and Bit Operations/Compare To Constant  relop=>=  const=130  OutDataTypeStr=boolean
  139-Compare : simulink/Logic and Bit Operations/Compare To Constant  relop=<=  const=139  OutDataTypeStr=boolean
  Constant11 : Constant
  Constant12 : Constant
  Constant13 : Constant  Value=0
  Constant14 : Constant  Value=0
  Constant26 : Constant  Value=4
  Logical Operator2 : Logic  AllPortsSameDT=off  OutDataTypeStr=boolean
  Product3 : Product
  Range_Lower : Switch  Criteria=u2 > Threshold  SaturateOnIntegerOverflow=off  InputSameDT=off
  Range_Upper : Switch  Criteria=u2 > Threshold  SaturateOnIntegerOverflow=off  InputSameDT=off
  Out1 : Outport
  wires:
  Input values/1 -> 139-Compare/1, 130+Compare/1
  Constant26/1 -> Product3/2
  Constant11/1 -> Range_Upper/1
  Constant14/1 -> Range_Lower/3
  Constant12/1 -> Range_Lower/1
  Logical Operator2/1 -> Product3/1
  130+Compare/1 -> Range_Upper/2
  139-Compare/1 -> Range_Lower/2
  Range_Lower/1 -> Logical Operator2/2
  Product3/1 -> Out1/1
  Range_Upper/1 -> Logical Operator2/1
  Constant13/1 -> Range_Upper/3

== system Integrated_Model/Subsystem2/Subsystem1/Subsystem/Systol_Ht2 ==
  Input value : Inport
  140+Compare : simulink/Logic and Bit Operations/Compare To Constant  relop=>=  const=140  OutDataTypeStr=boolean
  159-Compare : simulink/Logic and Bit Operations/Compare To Constant  relop=<=  const=159  OutDataTypeStr=boolean
  Constant15 : Constant
  Constant16 : Constant
  Constant17 : Constant  Value=0
  Constant18 : Constant  Value=0
  Constant27 : Constant  Value=5
  Logical Operator3 : Logic  AllPortsSameDT=off  OutDataTypeStr=boolean
  Product4 : Product
  Range_Lower : Switch  Criteria=u2 > Threshold  SaturateOnIntegerOverflow=off  InputSameDT=off
  Range_Upper : Switch  Criteria=u2 > Threshold  SaturateOnIntegerOverflow=off  InputSameDT=off
  Out1 : Outport
  wires:
  Constant16/1 -> Range_Lower/1
  159-Compare/1 -> Range_Lower/2
  Constant27/1 -> Product4/2
  Constant17/1 -> Range_Upper/3
  Input value/1 -> 140+Compare/1, 159-Compare/1
  Range_Upper/1 -> Logical Operator3/1
  Range_Lower/1 -> Logical Operator3/2
  Constant18/1 -> Range_Lower/3
  Logical Operator3/1 -> Product4/1
  140+Compare/1 -> Range_Upper/2
  Constant15/1 -> Range_Upper/1
  Product4/1 -> Out1/1

== system Integrated_Model/Subsystem2/Subsystem1/Subsystem/Systol_Htcrisis ==
  Input value : Inport
  180+Compare : simulink/Logic and Bit Operations/Compare To Constant  relop=>=  const=180  OutDataTypeStr=boolean
  260-Compare : simulink/Logic and Bit Operations/Compare To Constant  relop=<=  const=260  OutDataTypeStr=boolean
  Constant19 : Constant
  Constant20 : Constant
  Constant21 : Constant  Value=0
  Constant22 : Constant  Value=0
  Constant28 : Constant  Value=6
  Logical Operator4 : Logic  AllPortsSameDT=off  OutDataTypeStr=boolean
  Product5 : Product
  Range_Lower : Switch  Criteria=u2 > Threshold  SaturateOnIntegerOverflow=off  InputSameDT=off
  Range_Upper : Switch  Criteria=u2 > Threshold  SaturateOnIntegerOverflow=off  InputSameDT=off
  Out1 : Outport
  wires:
  Range_Lower/1 -> Logical Operator4/2
  Constant21/1 -> Range_Upper/3
  Constant22/1 -> Range_Lower/3
  260-Compare/1 -> Range_Lower/2
  180+Compare/1 -> Range_Upper/2
  Constant20/1 -> Range_Lower/1
  Range_Upper/1 -> Logical Operator4/1
  Logical Operator4/1 -> Product5/1
  Constant28/1 -> Product5/2
  Constant19/1 -> Range_Upper/1
  Input value/1 -> 180+Compare/1, 260-Compare/1
  Product5/1 -> Out1/1

== system Integrated_Model/Subsystem2/Subsystem1/Subsystem/Systol_Low ==
  Input_value : Inport
  100-Compare : simulink/Logic and Bit Operations/Compare To Constant  relop=<=  const=100  OutDataTypeStr=boolean
  90+compare : simulink/Logic and Bit Operations/Compare To Constant  relop=>=  const=90  OutDataTypeStr=boolean
  Constant1 : Constant
  Constant2 : Constant
  Constant23 : Constant
  Constant3 : Constant  Value=0
  Constant4 : Constant  Value=0
  Logical Operator : Logic  AllPortsSameDT=off  OutDataTypeStr=boolean
  Product : Product
  Range_Lower : Switch  Criteria=u2 > Threshold  SaturateOnIntegerOverflow=off  InputSameDT=off
  Range_Upper : Switch  Criteria=u2 > Threshold  SaturateOnIntegerOverflow=off  InputSameDT=off
  Out1 : Outport
  wires:
  Logical Operator/1 -> Product/1
  Constant3/1 -> Range_Upper/3
  Input_value/1 -> 100-Compare/1, 90+compare/1
  Range_Lower/1 -> Logical Operator/2
  Constant1/1 -> Range_Upper/1
  Constant23/1 -> Product/2
  Range_Upper/1 -> Logical Operator/1
  100-Compare/1 -> Range_Lower/2
  90+compare/1 -> Range_Upper/2
  Constant4/1 -> Range_Lower/3
  Constant2/1 -> Range_Lower/1
  Product/1 -> Out1/1

== system Integrated_Model/Subsystem2/Subsystem1/Subsystem/Systol_Normal ==
  Input value : Inport
  120Compare : simulink/Logic and Bit Operations/Compare To Constant  relop===  const=120  OutDataTypeStr=boolean
  Constant10 : Constant  Value=0
  Constant24 : Constant  Value=2
  Constant9 : Constant
  Product1 : Product
  Range_compare : Switch  Criteria=u2 > Threshold  SaturateOnIntegerOverflow=off  InputSameDT=off
  Out1 : Outport
  wires:
  Constant9/1 -> Range_compare/1
  120Compare/1 -> Range_compare/2
  Range_compare/1 -> Product1/1
  Constant24/1 -> Product1/2
  Product1/1 -> Out1/1
  Input value/1 -> 120Compare/1
  Constant10/1 -> Range_compare/3
